simulink model "mohinhhoa2020a"  (R2023b)
settings: Solver=VariableStepAuto  StartTime=0.0  StopTime=30  RelTol=1e-3
settings Model: Creator=ADMIN  LastModifiedBy=ACER
settings SolverCC: AlgebraicLoopSolver=TrustRegion

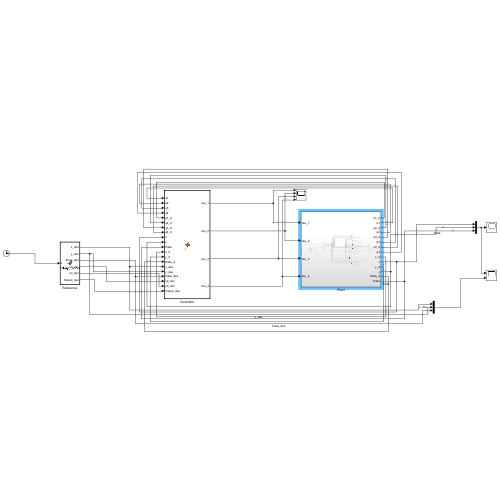
[thumbnail: Simulink's stored preview of the top-level diagram]
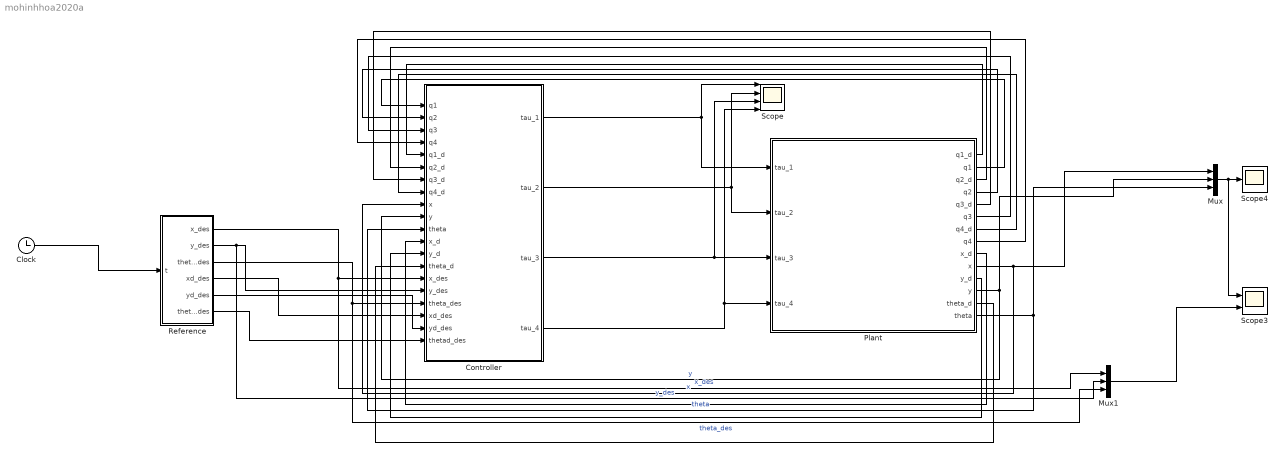
== system mohinhhoa2020a ==
  Clock : Clock
  Controller : MATLAB Function  TreatAsAtomicUnit=on
  Mux : Mux  Inputs=3
  Mux1 : Mux  Inputs=3
  Plant : Subsystem
  Reference : MATLAB Function  TreatAsAtomicUnit=on
  Scope : Scope  NumInputPorts=4
  Scope3 : Scope  NumInputPorts=2
  Scope4 : Scope
  wires:
  Clock/1 -> Reference/1(t)
  Reference/1(x_des) -> Mux1/1, Controller/15(x_des)  "x_des"
  Controller/1(tau_1) -> Plant/1(tau_1), Scope/1
  Plant/1(q1_d) -> Controller/5(q1_d)
  Plant/2(q1) -> Controller/1(q1)
  Plant/4(q2) -> Controller/2(q2)
  Plant/3(q2_d) -> Controller/6(q2_d)
  Plant/5(q3_d) -> Controller/7(q3_d)
  Plant/6(q3) -> Controller/3(q3)
  Plant/7(q4_d) -> Controller/8(q4_d)
  Plant/8(q4) -> Controller/4(q4)
  Plant/10(x) -> Mux/1, Controller/9(x)  "x"
  Plant/12(y) -> Mux/2, Controller/10(y)  "y"
  Plant/14(theta) -> Mux/3, Controller/11(theta)  "theta"
  Controller/2(tau_2) -> Plant/2(tau_2), Scope/2
  Controller/3(tau_3) -> Scope/3, Plant/3(tau_3)
  Controller/4(tau_4) -> Scope/4, Plant/4(tau_4)
  Mux/1 -> Scope3/1, Scope4/1
  Reference/3(theta_des) -> Mux1/3, Controller/17(theta_des)  "theta_des"
  Mux1/1 -> Scope3/2
  Reference/4(xd_des) -> Controller/18(xd_des)
  Reference/5(yd_des) -> Controller/19(yd_des)
  Reference/6(thetad_des) -> Controller/20(thetad_des)
  Plant/9(x_d) -> Controller/12(x_d)
  Plant/11(y_d) -> Controller/13(y_d)
  Plant/13(theta_d) -> Controller/14(theta_d)
  Reference/2(y_des) -> Mux1/2, Controller/16(y_des)  "y_des"

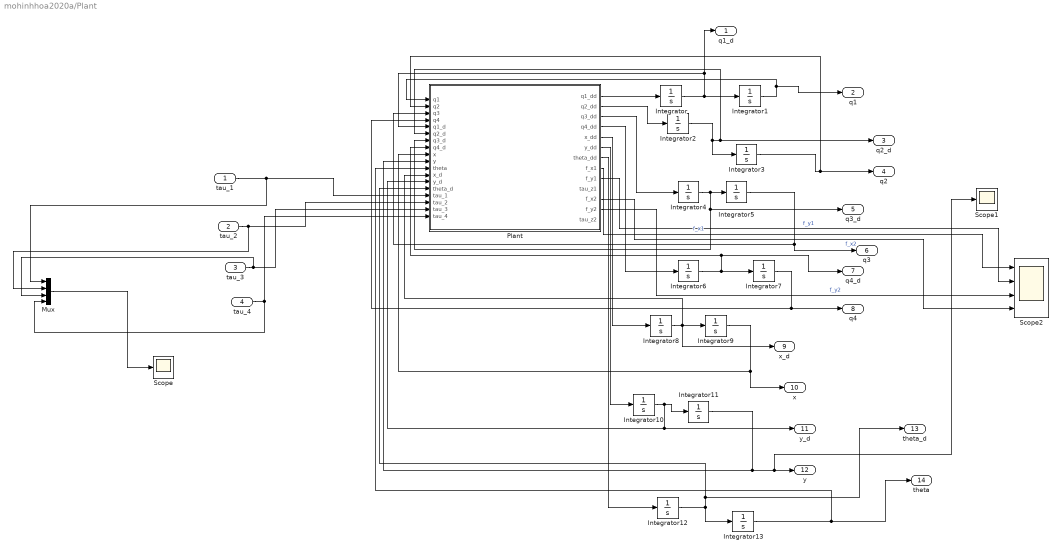
== system mohinhhoa2020a/Plant ==
  tau_1 : Inport
  tau_2 : Inport  Port=2
  tau_3 : Inport  Port=3
  tau_4 : Inport  Port=4
  Integrator{,2,4,6,8,10,12..13} (8 alike) : Integrator
  Integrator1 : Integrator  InitialCondition=1.4470
  Integrator11 : Integrator  InitialCondition=0.8
  Integrator3 : Integrator  InitialCondition=-1.6898
  Integrator5 : Integrator  InitialCondition=3.1353
  Integrator7 : Integrator  InitialCondition=-1.6898
  Integrator9 : Integrator  InitialCondition=1
  Mux : Mux
  Plant : MATLAB Function  TreatAsAtomicUnit=on
  Scope : Scope
  Scope1 : Scope
  Scope2 : Scope  NumInputPorts=4
  q1_d : Outport
  q1 : Outport  Port=2
  q2_d : Outport  Port=3
  q2 : Outport  Port=4
  q3_d : Outport  Port=5
  q3 : Outport  Port=6
  q4_d : Outport  Port=7
  q4 : Outport  Port=8
  x_d : Outport  Port=9
  x : Outport  Port=10
  y_d : Outport  Port=11
  y : Outport  Port=12
  theta_d : Outport  Port=13
  theta : Outport  Port=14
  wires:
  tau_1/1 -> Mux/1, Plant/15(tau_1)
  Plant/1(q1_dd) -> Integrator/1
  Integrator/1 -> q1_d/1, Plant/5(q1_d), Integrator1/1
  Integrator1/1 -> q1/1, Plant/1(q1)
  Plant/2(q2_dd) -> Integrator2/1
  Integrator2/1 -> Plant/6(q2_d), q2_d/1, Integrator3/1
  Integrator3/1 -> q2/1, Plant/2(q2)
  Plant/3(q3_dd) -> Integrator4/1
  Integrator4/1 -> Plant/7(q3_d), q3_d/1, Integrator5/1
  Integrator5/1 -> q3/1, Plant/3(q3)
  Plant/4(q4_dd) -> Integrator6/1
  Integrator6/1 -> Plant/8(q4_d), q4_d/1, Integrator7/1
  Integrator7/1 -> q4/1, Plant/4(q4)
  Plant/5(x_dd) -> Integrator8/1
  Integrator8/1 -> x_d/1, Plant/12(x_d), Integrator9/1
  Integrator9/1 -> Plant/9(x), x/1
  Plant/6(y_dd) -> Integrator10/1
  Integrator10/1 -> y_d/1, Plant/13(y_d), Integrator11/1
  Integrator11/1 -> Scope1/1, y/1, Plant/10(y)
  Plant/7(theta_dd) -> Integrator12/1
  Integrator12/1 -> Plant/14(theta_d), theta_d/1, Integrator13/1
  Integrator13/1 -> Plant/11(theta), theta/1
  tau_2/1 -> Mux/2, Plant/16(tau_2)
  tau_3/1 -> Mux/3, Plant/17(tau_3)
  tau_4/1 -> Mux/4, Plant/18(tau_4)
  Mux/1 -> Scope/1
  Plant/8(f_x1) -> Scope2/1  "f_x1"
  Plant/9(f_y1) -> Scope2/2  "f_y1"
  Plant/11(f_x2) -> Scope2/4  "f_x2"
  Plant/12(f_y2) -> Scope2/3  "f_y2"

== matlab function mohinhhoa2020a/Reference ==
  data: t input; x_des output; y_des output; theta_des output; xd_des output; yd_des output; thetad_des output
function [x_des,y_des,theta_des,xd_des,yd_des,thetad_des]  = Trajectory_Generator(t)
   
Start_Val = [1;   0.8 ;  0];       % x=0, y=1m,  ngang
End_Val   = [1;  1.45; 0.8];     %  [1;  1.45; 0.8];
                                 %[1.2;  0.55; 0] chỉ tune được xy 
T_finish=30;
alpha=0.1; 
    % 1. Tính vector chênh lệch (Target - Start)
    Diff = End_Val - Start_Val;

    % 2. Kiểm tra thời gian
    if t >= T_finish
        % Nếu hết giờ, giữ nguyên vị trí đích, vận tốc = 0
        xc_des = End_Val;
        vc_des = zeros(size(Start_Val));
    else
        % 3. Tính hệ số hàm mũ (Exponential term)
        % Công thức bài báo: profile = e^(-alpha * t^2)
        exp_term = exp(-alpha * t^2);
        
        % 4. Tính Vị trí mong muốn (Theo Eq 47)
        % x(t) = x_f - (x_f - x_i) * e^(-alpha*t^2)
        xc_des = End_Val - Diff * exp_term;
        
        % 5. Tính Vận tốc mong muốn (Đạo hàm của vị trí)
        % v(t) = (x_f - x_i) * 2 * alpha * t * e^(-alpha*t^2)
        vc_des = Diff * (2 * alpha * t) * exp_term;
    end

x_des = xc_des(1);
y_des = xc_des(2);
theta_des = xc_des(3);
xd_des = vc_des(1);
yd_des = vc_des(2);
thetad_des = vc_des(3);

== matlab function mohinhhoa2020a/Controller ==
  data: q1 input; tau_1 output; q2 input; q3 input; q4 input; q1_d input; q2_d input; q3_d input; q4_d input; x input; y input; theta input; x_d input; y_d input; theta_d input; x_des input; tau_2 output; tau_3 output; tau_4 output; y_des input; theta_des input; xd_des input; yd_des input; thetad_des input
function [tau_1,tau_2,tau_3,tau_4] = fcn(q1,q2,q3,q4,q1_d,q2_d,q3_d,q4_d,x,y,theta,x_d,y_d,theta_d,x_des,y_des,theta_des,xd_des,yd_des,thetad_des)
%%%%%%%%%%%%%%%%%%%%%%%%%%%%%%%%%%%%%%Modeling%%%%%%%%%%%%%%%%%%%%%%%%%%%%%%%%%%%
%%%% Các tham số:
g=9.81;
m = 5;
a = 0.2; b = 0.2;
L=0.2;
l1=1;
l2=0.8;
l3=l1;
l4=l2;
m1=1.5;
m2=1;
m3=m1;
m4=m2;
I1=(1/12)*m1*(l1^2);
I2=(1/12)*m2*(l2^2);
I3=I1;
I4=I2;
%%%%% Mô hình cánh tay 
%  Vector q_d
q_d = [q1_d;q2_d;q3_d;q4_d];
%Ma trận M
M_11_b = I3 + I4 + (l3^2*m3)/4 + l3^2*m4 + (l4^2*m4)/4 + l3*l4*m4*cos(q4);
M_12_b = (m4*l4^2)/4 + (l3*m4*cos(q4)*l4)/2 + I4;
M_21_b = (m4*l4^2)/4 + (l3*m4*cos(q4)*l4)/2 + I4;
M_22_b = (m4*l4^2)/4 + I4;
M_B = [M_11_b, M_12_b;
    M_21_b, M_22_b];
M_11_a = I1 + I2 + (l1^2*m1)/4 + l1^2*m2 + (l2^2*m2)/4 + l1*l2*m2*cos(q2);
M_12_a = (m2*l2^2)/4 + (l1*m2*cos(q2)*l2)/2 + I2;
M_21_a = (m2*l2^2)/4 + (l1*m2*cos(q2)*l2)/2 + I2;
M_22_a = (m2*l2^2)/4 + I2;
M_A = [M_11_a, M_12_a;
    M_21_a, M_22_a];
M = [M_A zeros(2,2);
    zeros(2,2) M_B];
%Ma trận C
C_11_a = -(q2_d*l1*l2*m2*sin(q2))/2;
C_12_a = -(l1*l2*m2*sin(q2)*(q1_d + q2_d))/2;
C_21_a = (q1_d*l1*l2*m2*sin(q2))/2;
C_22_a= 0;
C_A = [C_11_a, C_12_a;
    C_21_a, C_22_a];
C_11_b = -(q4_d*l3*l4*m4*sin(q4))/2;
C_12_b = -(l3*l4*m4*sin(q4)*(q3_d + q4_d))/2;
C_21_b = (q3_d*l3*l4*m4*sin(q4))/2;
C_22_b= 0;
C_B = [C_11_b, C_12_b;
    C_21_b, C_22_b];
C = [C_A zeros(2,2);
    zeros(2,2) C_B];
%Ma trận k
k_1_a = (g*(l1*m1*cos(q1) + 2*l1*m2*cos(q1) + l2*m2*cos(q1 + q2)))/2;
k_2_a = (g*l2*m2*cos(q1 + q2))/2;
k_1_b = (g*(l3*m3*cos(q3) + 2*l3*m4*cos(q3) + l4*m4*cos(q3 + q4)))/2;
k_2_b = (g*l4*m4*cos(q3 + q4))/2;
k = [k_1_a;k_2_a;k_1_b;k_2_b];
% Ma trận Jacobian (Sửa thành 3x2)
% Hàng 1: Vx, Hàng 2: Vy, Hàng 3: Omega
J_A = [-l1*sin(q1)-l2*sin(q1+q2),  -l2*sin(q1+q2);
        l1*cos(q1)+l2*cos(q1+q2),   l2*cos(q1+q2);
        1,                          1]; % Thêm hàng này: Omega = q1_dot + q2_dot

J_d_A = [-q1_d*(l2*cos(q1 + q2) + l1*cos(q1)) - q2_d*l2*cos(q1 + q2), -l2*cos(q1 + q2)*(q1_d + q2_d);
         -q1_d*(l2*sin(q1 + q2) + l1*sin(q1)) - q2_d*l2*sin(q1 + q2), -l2*sin(q1 + q2)*(q1_d + q2_d);
          0,                                                           0]; % Đạo hàm của hằng số 1 là 0

J_B = [-l3*sin(q3)-l4*sin(q3+q4),  -l4*sin(q3+q4);
        l3*cos(q3)+l4*cos(q3+q4),   l4*cos(q3+q4);
        1,                          1]; % Thêm hàng Omega cho tay 2

J_d_B = [-q3_d*(l4*cos(q3 + q4) + l3*cos(q3)) - q4_d*l4*cos(q3 + q4), -l4*cos(q3 + q4)*(q3_d + q4_d);
         -q3_d*(l4*sin(q3 + q4) + l3*sin(q3)) - q4_d*l4*sin(q3 + q4), -l4*sin(q3 + q4)*(q3_d + q4_d);
          0,                                                           0];

% Ghép Jacobian tổng (Bây giờ là 6x4)
J = [J_A, zeros(3,2);
     zeros(3,2), J_B];
J_d = [J_d_A, zeros(3,2);
       zeros(3,2), J_d_B];
%%%%% Mô hình vật thể
Izz = (m/12)*((a^2)+(b^2));
Mc = diag([m, m, Izz]);
bc = [0;0;0];
kc = [0; -m*g; 0];
% Ma trận Grasp A_T (3x4)
    % 2. Tính cánh tay đòn trong hệ World (Quan trọng!)
    % r_body: Vector từ tâm vật đến điểm chạm (Hằng số)
    r1_body = [-L/2; 0]; 
    r2_body = [ L/2; 0];
    % Ma trận quay
    R = [cos(theta), -sin(theta);
         sin(theta),  cos(theta)];
         
    % Quay vector r ra hệ World
    r1_world = R * r1_body; % = [r1x_w; r1y_w]
    r2_world = R * r2_body; % = [r2x_w; r2y_w]
   % A_T1 cho tay 1:
% Fx = fx1
% Fy = fy1
% Tau = tau1 + (rx * fy1 - ry * fx1)
    A_T1 = [1,            0,            0; 
        0,            1,            0; 
       -r1_world(2),  r1_world(1),  1]; % Số 1 ở cuối là để truyền Tau1 trực tiếp

% A_T2 cho tay 2:
A_T2 = [1,            0,            0; 
        0,            1,            0; 
       -r2_world(2),  r2_world(1),  1];

% Ghép lại
A_T = [A_T1, A_T2];
% Tính lực f chuyển về dạng Ax=b để tránh dùng inv tính nghịch đảo
J_T = J.';
%%%%%%%%%%%%%%%%%%%%%%%%%%%%%%%%%%%Controller%%%%%%%%%%%%%%%%%%%%%%%%%%%%%%%%%%%%
% Tính toán tau_g (Compensation)
F_lift_total = -kc; % = [0; m*g; 0]
%%% Chia đôi lực nâng cho 2 tay (Load Balancing đơn giản)
    F_lift_distributed = [F_lift_total/2; F_lift_total/2]; % Vector 6x1
A_hat_T = blkdiag(A_T1, A_T2); % Kích thước 6x6
Fk = pinv(A_hat_T)*F_lift_distributed;
tau_g = k + J_T*Fk;
% Tính toán tau_m (Motion Control)
% tau_p:
x_c = [x;y;theta];
xc_des = [x_des;y_des;theta_des];
delta_x = xc_des - x_c;
%%%%%%%%%%%%%%%%%Tunning%%%%%%%%%%%%%%%%%%
Kp=diag([50,50, 0]); %[50,50, 0] ; [50,5, 0]
Dm= 1 * eye(4); %1
Kv=diag([10,10, 0]); %[10,10, 0] ; [0,10, 0]
%%%%%%%%%%%%%%%%%%%%%%%%%%%%%%%%%%%%%%%%%
F_P = pinv(A_T)*(Kp*delta_x);
tau_p = J_T*F_P;
% tau_v :
vc_des = [xd_des;yd_des;thetad_des];
v_c = [x_d;y_d;theta_d];
delta_v = vc_des-v_c;
F_D = pinv(A_T)*(Kv*vc_des);
tau_v = J_T*F_D - Dm*q_d;

% tau_m
tau_m = (tau_v+tau_p) ;
% Tính toán tau_s (Force Control)
% Ma trận Nullspace trực chuẩn (Orthonormal)
Q1 = eye(4); %%%%%%%%%%%%Tunning
Q2 = 1000 * eye(6);  %%%%%%%%%%%%%Tunning
val = 1/sqrt(2);
A_tilde_c_T = [ val,  0,    0;
                0,    val,  0;
                0,    0,    val;
               -val,  0,    0;
                0,   -val,  0;
                0,    0,   -val ];
A_tilde_c = A_tilde_c_T.';
%%%%thành phần lực:
% 1. eta (Lực bắt buộc để nâng vật)
eta = Fk; 

% 2. fc_des (Lực mong muốn tổng hợp)
% Đặt lực nén mong muốn: 20N (Ví dụ)
target_squeeze = [0; 20; 0]; 
f_squeeze_vec = A_tilde_c_T * target_squeeze;
% Tổng hợp
fc_des = eta + f_squeeze_vec;
Df = J_T*A_tilde_c_T;
Df_T = Df.';
xi_1 = Df_T*Q1*Df + A_tilde_c*Q2*A_tilde_c_T;
xi_2 = (Df_T*Q1*(tau_m+tau_g)+A_tilde_c*Q2*(fc_des-eta));
xi = -xi_1\xi_2;
tau_s = J_T*(A_hat_T\(A_tilde_c_T*xi));
% Tổng tín hiệu:
tau = tau_m + tau_s+ tau_g;
tau_1 = tau(1);
tau_2 = tau(2);
tau_3 = tau(3);
tau_4 = tau(4);

== matlab function mohinhhoa2020a/Plant/Plant ==
  data: q1 input; q1_dd output; q2 input; q3 input; q4 input; q1_d input; q2_d input; q3_d input; q4_d input; q2_dd output; x input; y input; theta input; x_d input; y_d input; theta_d input; tau_1 input; q3_dd output; q4_dd output; x_dd output; y_dd output; theta_dd output; tau_2 input; tau_3 input; tau_4 input; f_x1 output; f_y1 output; tau_z1 output; f_x2 output; f_y2 output; tau_z2 output
function [q1_dd,q2_dd,q3_dd,q4_dd,x_dd,y_dd,theta_dd,f_x1,f_y1,tau_z1,f_x2,f_y2,tau_z2]  = fcn(q1,q2,q3,q4,q1_d,q2_d,q3_d,q4_d,x,y,theta,x_d,y_d,theta_d,tau_1,tau_2,tau_3,tau_4)
tau = [tau_1;tau_2;tau_3;tau_4];
%%%% Các tham số:
g=9.81;
m = 5;
a = 0.2; b = 0.2;
L=0.2;
l1=1;
l2=0.8;
l3=l1;
l4=l2;
m1=1.5;
m2=1;
m3=m1;
m4=m2;
I1=(1/12)*m1*(l1^2);
I2=(1/12)*m2*(l2^2);
I3=I1;
I4=I2;
%%%%% Mô hình cánh tay 
%  Vector q_d
q_d = [q1_d;q2_d;q3_d;q4_d];
%Ma trận M
M_11_b = I3 + I4 + (l3^2*m3)/4 + l3^2*m4 + (l4^2*m4)/4 + l3*l4*m4*cos(q4);
M_12_b = (m4*l4^2)/4 + (l3*m4*cos(q4)*l4)/2 + I4;
M_21_b = (m4*l4^2)/4 + (l3*m4*cos(q4)*l4)/2 + I4;
M_22_b = (m4*l4^2)/4 + I4;
M_B = [M_11_b, M_12_b;
    M_21_b, M_22_b];
M_11_a = I1 + I2 + (l1^2*m1)/4 + l1^2*m2 + (l2^2*m2)/4 + l1*l2*m2*cos(q2);
M_12_a = (m2*l2^2)/4 + (l1*m2*cos(q2)*l2)/2 + I2;
M_21_a = (m2*l2^2)/4 + (l1*m2*cos(q2)*l2)/2 + I2;
M_22_a = (m2*l2^2)/4 + I2;
M_A = [M_11_a, M_12_a;
    M_21_a, M_22_a];
M = [M_A zeros(2,2);
    zeros(2,2) M_B];
%Ma trận C
C_11_a = -(q2_d*l1*l2*m2*sin(q2))/2;
C_12_a = -(l1*l2*m2*sin(q2)*(q1_d + q2_d))/2;
C_21_a = (q1_d*l1*l2*m2*sin(q2))/2;
C_22_a= 0;
C_A = [C_11_a, C_12_a;
    C_21_a, C_22_a];
C_11_b = -(q4_d*l3*l4*m4*sin(q4))/2;
C_12_b = -(l3*l4*m4*sin(q4)*(q3_d + q4_d))/2;
C_21_b = (q3_d*l3*l4*m4*sin(q4))/2;
C_22_b= 0;
C_B = [C_11_b, C_12_b;
    C_21_b, C_22_b];
C = [C_A, zeros(2,2);
    zeros(2,2), C_B];
%Ma trận k
k_1_a = (g*(l1*m1*cos(q1) + 2*l1*m2*cos(q1) + l2*m2*cos(q1 + q2)))/2;
k_2_a = (g*l2*m2*cos(q1 + q2))/2;
k_1_b = (g*(l3*m3*cos(q3) + 2*l3*m4*cos(q3) + l4*m4*cos(q3 + q4)))/2;
k_2_b = (g*l4*m4*cos(q3 + q4))/2;
k = [k_1_a;k_2_a;k_1_b;k_2_b];
% Ma trận Jacobian (Sửa thành 3x2)
% Hàng 1: Vx, Hàng 2: Vy, Hàng 3: Omega
J_A = [-l1*sin(q1)-l2*sin(q1+q2),  -l2*sin(q1+q2);
        l1*cos(q1)+l2*cos(q1+q2),   l2*cos(q1+q2);
        1,                          1]; % Thêm hàng này: Omega = q1_dot + q2_dot

J_d_A = [-q1_d*(l2*cos(q1 + q2) + l1*cos(q1)) - q2_d*l2*cos(q1 + q2), -l2*cos(q1 + q2)*(q1_d + q2_d);
         -q1_d*(l2*sin(q1 + q2) + l1*sin(q1)) - q2_d*l2*sin(q1 + q2), -l2*sin(q1 + q2)*(q1_d + q2_d);
          0,                                                           0]; % Đạo hàm của hằng số 1 là 0

J_B = [-l3*sin(q3)-l4*sin(q3+q4),  -l4*sin(q3+q4);
        l3*cos(q3)+l4*cos(q3+q4),   l4*cos(q3+q4);
        1,                          1]; % Thêm hàng Omega cho tay 2

J_d_B = [-q3_d*(l4*cos(q3 + q4) + l3*cos(q3)) - q4_d*l4*cos(q3 + q4), -l4*cos(q3 + q4)*(q3_d + q4_d);
         -q3_d*(l4*sin(q3 + q4) + l3*sin(q3)) - q4_d*l4*sin(q3 + q4), -l4*sin(q3 + q4)*(q3_d + q4_d);
          0,                                                           0];

% Ghép Jacobian tổng (Bây giờ là 6x4)
J = [J_A, zeros(3,2);
     zeros(3,2), J_B];

J_d = [J_d_A, zeros(3,2);
       zeros(3,2), J_d_B];
%%%%% Mô hình vật thể
Izz = (m/12)*((a^2)+(b^2));
Mc = diag([m, m, Izz]);
bc = [0;0;0];
kc = [0; -m*g; 0];
% Ma trận Grasp A_T (3x4)
    % 2. Tính cánh tay đòn trong hệ World (Quan trọng!)
    % r_body: Vector từ tâm vật đến điểm chạm (Hằng số)
    r1_body = [-L/2; 0]; 
    r2_body = [ L/2; 0];
    % Ma trận quay
    R = [cos(theta), -sin(theta);
         sin(theta),  cos(theta)];
         
    % Quay vector r ra hệ World
    r1_world = R * r1_body; % = [r1x_w; r1y_w]
    r2_world = R * r2_body; % = [r2x_w; r2y_w]
   % A_T1 cho tay 1:
% Fx = fx1
% Fy = fy1
% Tau = tau1 + (rx * fy1 - ry * fx1)
    A_T1 = [1,            0,            0; 
        0,            1,            0; 
       -r1_world(2),  r1_world(1),  1]; % Số 1 ở cuối là để truyền Tau1 trực tiếp

% A_T2 cho tay 2:
A_T2 = [1,            0,            0; 
        0,            1,            0; 
       -r2_world(2),  r2_world(1),  1];

% Ghép lại
A_T = [A_T1, A_T2];
% Tính lực f chuyển về dạng Ax=b để tránh dùng inv tính nghịch đảo
J_T = J.';
A = A_T.';
% Tính toán bias gia tốc (acc)
% a_linear = -omega^2 * r (cho x và y)
% a_angular = 0 (cho theta, vì kẹp cứng không thay đổi góc tương đối)
a1 = [-(theta_d^2) * r1_world; 0]; % Thêm 0 vào cuối -> vector 3x1
a2 = [-(theta_d^2) * r2_world; 0]; % Thêm 0 vào cuối -> vector 3x1
    
    % Ghép lại thành vector bias tổng cho cả 2 điểm chạm
    acc = [a1;a2];
Left_Mat = [M,      zeros(4,3),       J_T; 
                zeros(3,4),      Mc,     -A_T;
                J,      -A,     zeros(6,6)];
Right_Vec = [tau-C*q_d-k;(bc+kc);-J_d*q_d+acc];
Solution = Left_Mat \ Right_Vec;
  % Trích xuất kết quả
   % Gia tốc khớp
    q_dd    = Solution(1:4);
    q1_dd = q_dd(1);
    q2_dd = q_dd(2);
    q3_dd = q_dd(3);
    q4_dd = q_dd(4);
    % Gia tốc vật
    alpha_c = Solution(5:7);
    x_dd = alpha_c(1);
    y_dd = alpha_c(2);
    theta_dd = alpha_c(3);
    % Lực tiếp xúc (Bây giờ f có 6 thành phần: fx1, fy1, tau1, fx2, fy2, tau2)
    f_x1       = Solution(8);
    f_y1 = Solution(9);
    tau_z1 = Solution(10);
    f_x2       = Solution(11);
    f_y2 = Solution(12);
    tau_z2 = Solution(13);
